simulink model "rths_tp5b707349_fd62_4425_8506_d65370c4e4cc"  (R2025b)
settings: Solver=ode4  StartTime=0.0  StopTime=40  FixedStep=dt  RelTol=1e-3
model workspace (MAT data in the model file):
  A1 = [0 0 0 0 0 0 0 0 0 0 0 0 ... (900 elements, 30x30)]
  A2 = [0  0  0  0  0  1  0  0  0  0; 0  0  0  0  0  0  1  0  0  0; 0  0  0  0  0  0  0  1  0  0; 0  0  0  0  0  0  0  0  1  0; 0  0  0  0  0  0  0  0  0  1; -6205.60302527  1405.13447498  -1011.0594463  369.077338518  661.723706661  -9.52439456266  1.85806890853  -1.33696678524  0.488046617428  0.875025321263; 1645.79621993  -1248.4516031  -584.204769511  -445.124925438  -14.757742624  2.17630614043  -2.96934300253  -0.772518743063  -0.588607566818  -0.019514788953; -31811.1306157  -18833.1920383  -40326.5026179  -9876.3778695  -4570.38300075  -42.0652071349  -24.9039285548  -54.6439071739  -13.0599533176  -6.04361127351; 42386.9190877  -43864.1201358  -10414.2582056  -47790.9085772  -9989.44252289  56.0500207544  -58.003386349  -13.7712152978  -64.514407742  -13.2094635039; 32393.8023142  -24338.2549642  -6423.44335823  -10363.3236005  -23491.5690202  42.835698633  -32.1835067334  -8.49399157318  -13.7038623093  -32.3823605019]
  A3 = [0 0 0 0 0 0 0 0 -6465.93985904 1514.25007638 -29949.4995057 42366.3776755 ... (256 elements, 16x16)]
  B1 = [0  0  0  0  0  0  0  0  0  0  0  0  0  0  0; 0  0  0  0  0  0  0  0  0  0  0  0  0  0  0; 0  0  0  0  0  0  0  0  0  0  0  0  0  0  0; 0  0  0  0  0  0  0  0  0  0  0  0  0  0  0; 0  0  0  0  0  0  0  0  0  0  0  0  0  0  0; 0  0  0  0  0  0  0  0  0  0  0  0  0  0  0; 0  0  0  0  0  0  0  0  0  0  0  0  0  0  0; 0  0  0  0  0  0  0  0  0  0  0  0  0  0  0; 0  0  0  0  0  0  0  0  0  0  0  0  0  0  0; 0  0  0  0  0  0  0  0  0  0  0  0  0  0  0; 0  0  0  0  0  0  0  0  0  0  0  0  0  0  0; 0  0  0  0  0  0  0  0  0  0  0  0  0  0  0; 0  0  0  0  0  0  0  0  0  0  0  0  0  0  0; 0  0  0  0  0  0  0  0  0  0  0  0  0  0  0; 0  0  0  0  0  0  0  0  0  0  0  0  0  0  0; 0.000162210458758  0  0  0  0  0  0  0  0  0  0  0  0  0  0; 0  0.0195741403137  0  0  0  0  0  0  0  0  0  0  0  0  0; 0  0  0.0147303099554  0  0  0  0  0  0  0  0  0  0  0  0; 0  0  0  0.0147303099554  0  0  0  0  0  0  0  0  0  0  0; 0  0  0  0  0.0195741403137  0  0  0  0  0  0  0  0  0  0; 0  0  0  0  0  0.000162210458758  0  0  0  0  0  0  0  0  0; 0  0  0  0  0  0  0.0195741403137  0  0  0  0  0  0  0  0; 0  0  0  0  0  0  0  0.0147303099554  0  0  0  0  0  0  0; 0  0  0  0  0  0  0  0  0.0147303099554  0  0  0  0  0  0; 0  0  0  0  0  0  0  0  0  0.0195741403137  0  0  0  0  0; 0  0  0  0  0  0  0  0  0  0  0.000162210458758  0  0  0  0; 0  0  0  0  0  0  0  0  0  0  0  0.0195741403137  0  0  0; 0  0  0  0  0  0  0  0  0  0  0  0  0.0147303099554  0  0; 0  0  0  0  0  0  0  0  0  0  0  0  0  0.0147303099554  0; 0  0  0  0  0  0  0  0  0  0  0  0  0  0  0.0195741403137]
  B2 = [0  0  0  0  0; 0  0  0  0  0; 0  0  0  0  0; 0  0  0  0  0; 0  0  0  0  0; 0.000118340590374  -1.86972521181e-05  0.000266543526966  5.89063151674e-06  -0.000245845661968; -1.86972521181e-05  0.000140891598863  0.000147127517349  -9.46880125041e-06  -0.000148631232173; 0.000266543526966  0.000147127517349  0.012662466011  0.000116184727057  0.00167924700146; 5.89063151674e-06  -9.46880125041e-06  0.000116184727057  0.0146505342635  -7.75211989033e-06; -0.000245845661968  -0.000148631232173  0.00167924700146  -7.75211989033e-06  0.0131090855897]
  B3 = [0  0  0  0  0  0  0  0; 0  0  0  0  0  0  0  0; 0  0  0  0  0  0  0  0; 0  0  0  0  0  0  0  0; 0  0  0  0  0  0  0  0; 0  0  0  0  0  0  0  0; 0  0  0  0  0  0  0  0; 0  0  0  0  0  0  0  0; 0.000153222079678  -1.38864775191e-06  6.80539052363e-06  1.64914321893e-05  -2.57137705377e-05  0.00857679801195  -0.000293449983094  0.000726097409968; -1.38864775191e-06  0.000149515144127  1.93940221838e-05  -5.12172676809e-06  -3.82827328132e-05  0.00423910351833  -0.000212205388444  0.000534478402469; 6.80539052363e-06  1.93940221838e-05  0.0146353780333  5.09760170252e-06  8.11087485506e-05  -0.0644103990989  -0.000816445152791  5.37981551207e-05; 1.64914321893e-05  -5.12172676809e-06  5.09760170252e-06  0.0146828972607  1.89184773836e-05  0.00301816330771  0.0037908129159  -0.00354316274617; -2.57137705377e-05  -3.82827328132e-05  8.11087485506e-05  1.89184773836e-05  0.0145571946627  0.0536495512827  -0.00848725124143  0.00847023294881; 0.00857679801195  0.00423910351833  -0.0644103990989  0.00301816330771  0.0536495512827  2.11717274554  -0.0520147420295  0.0899270581681; -0.000293449983094  -0.000212205388444  -0.000816445152791  0.0037908129159  -0.00848725124143  -0.0520147420295  1.00698052503  -0.00826432567244; 0.000726097409968  0.000534478402469  5.37981551207e-05  -0.00354316274617  0.00847023294881  0.0899270581681  -0.00826432567244  1.01153242275]
  C1 = [1  0  0  0  0  0  0  0  0  0  0  0  0  0  0  0  0  0  0  0  0  0  0  0  0  0  0  0  0  0; 0  0  0  0  0  1  0  0  0  0  0  0  0  0  0  0  0  0  0  0  0  0  0  0  0  0  0  0  0  0; 0  0  0  0  0  0  0  0  0  0  1  0  0  0  0  0  0  0  0  0  0  0  0  0  0  0  0  0  0  0]
  C2 = [1  0  0  0  0  0  0  0  0  0; 0.719397421364  0.455029805905  -0.0548687646055  0.00094719287358  0.0504515218309  0  0  0  0  0; 0  1  0  0  0  0  0  0  0  0]
  C3 = [1  0  0  0  0  0  0  0  0  0  0  0  0  0  0  0; 0.719397421364  0.455029805905  -0.0548687646055  0.00094719287358  0.0504515218309  -0.0115996183931  0.000450409849156  -0.00105854789448  0  0  0  0  0  0  0  0; 0  1  0  0  0  0  0  0  0  0  0  0  0  0  0  0]
  D1 = [0  0  0  0  0  0  0  0  0  0  0  0  0  0  0; 0  0  0  0  0  0  0  0  0  0  0  0  0  0  0; 0  0  0  0  0  0  0  0  0  0  0  0  0  0  0]
  D2 = [0  0  0  0  0; 0  0  0  0  0; 0  0  0  0  0]
  D3 = [0  0  0  0  0  0  0  0; 0  0  0  0  0  0  0  0; 0  0  0  0  0  0  0  0]
  cb_force = [10599.793839; 8970.01227322; -338.256639094; 5.83928361236; 311.025085664; -71.5096824327; 2.7767004212; -6.52576845281]
  dt = 0.0009765625
  excitation_input = [0 0.0009765625 0.001953125 0.0029296875 0.00390625 0.0048828125 0.005859375 0.0068359375 0.0078125 0.0087890625 0.009765625 0.0107421875 ... (81922 elements, 40961x2)]
  full_force = [6164.83060128; 0; 0; 0; 0; 6164.83060128; 0; 0; 0; 0; 6164.83060128; 0; 0; 0; 0]
  guyan_force = [10599.793839; 8970.01227322; -338.256639094; 5.83928361236; 311.025085664]
settings Model: Creator=lenovo  LastModifiedBy=lenovo
settings DataIOCC: SaveOutput=off  SignalLogging=off  SaveTime=off

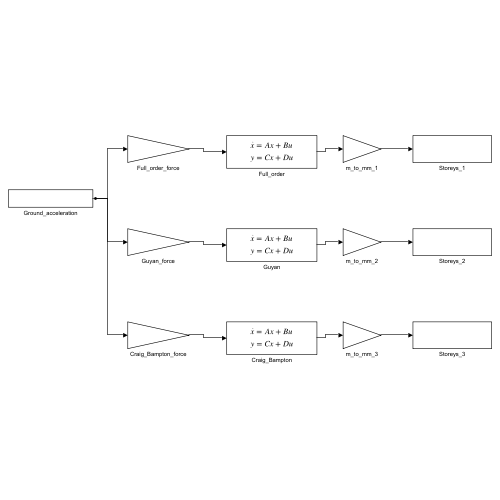
[thumbnail: Simulink's stored preview of the top-level diagram]
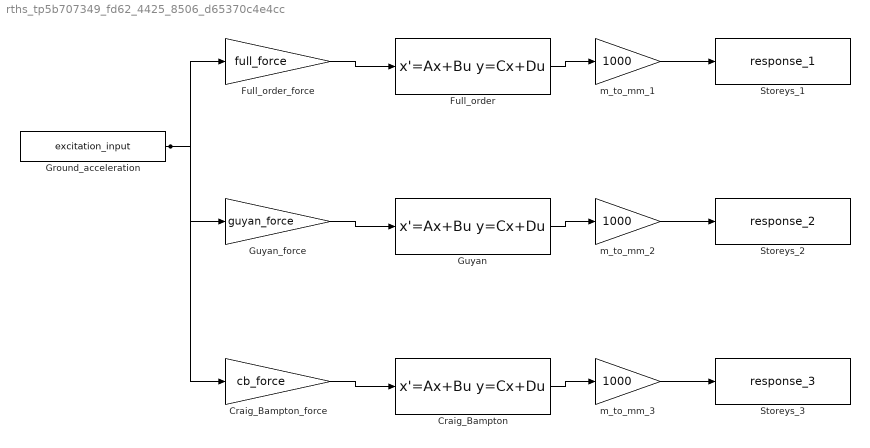
== system rths_tp5b707349_fd62_4425_8506_d65370c4e4cc ==
  Craig_Bampton : StateSpace  A=A3  B=B3  C=C3  D=D3  InitialCondition=0
  Craig_Bampton_force : Gain  Gain=cb_force
  Full_order : StateSpace  A=A1  B=B1  C=C1  D=D1  InitialCondition=0
  Full_order_force : Gain  Gain=full_force
  Ground_acceleration : FromWorkspace  VariableName=excitation_input  OutputAfterFinalValue=Holding final value
  Guyan : StateSpace  A=A2  B=B2  C=C2  D=D2  InitialCondition=0
  Guyan_force : Gain  Gain=guyan_force
  Storeys_1 : ToWorkspace  VariableName=response_1  SaveFormat=Timeseries  SampleTime=-1
  Storeys_2 : ToWorkspace  VariableName=response_2  SaveFormat=Timeseries  SampleTime=-1
  Storeys_3 : ToWorkspace  VariableName=response_3  SaveFormat=Timeseries  SampleTime=-1
  m_to_mm_1 : Gain  Gain=1000
  m_to_mm_2 : Gain  Gain=1000
  m_to_mm_3 : Gain  Gain=1000
  wires:
  Ground_acceleration/1 -> Full_order_force/1, Guyan_force/1, Craig_Bampton_force/1
  Full_order_force/1 -> Full_order/1
  Full_order/1 -> m_to_mm_1/1
  m_to_mm_1/1 -> Storeys_1/1
  Guyan_force/1 -> Guyan/1
  Guyan/1 -> m_to_mm_2/1
  m_to_mm_2/1 -> Storeys_2/1
  Craig_Bampton_force/1 -> Craig_Bampton/1
  Craig_Bampton/1 -> m_to_mm_3/1
  m_to_mm_3/1 -> Storeys_3/1
